simulink model "SimulinkOnramp"  (R2021a)
settings: Solver=VariableStepAuto  StartTime=0.0  StopTime=10.0  RelTol=1e-3
StartFcn:
  | learning.simulink.modelCallbacks.startFunction(gcs)
StopFcn:
  | learning.simulink.modelCallbacks.stopFunction(gcs)
model workspace (MAT data in the model file):
  courseObject.course = 'simulink'
  courseObject.chapter = 9
  courseObject.lesson = 1
  courseObject.section = 2
  courseObject.task = 1
  t_ans = [0; 0.25; 0.5; 0.75; 1; 1.25; 1.5; 1.75; 2; 2.25; 2.5; 2.75; 3; 3.25; 3.5; 3.75; 4; 4.25; 4.5; 4.75; 5; 5.25; 5.5; 5.75; 6; 6.25; 6.5; 6.75; 7; 7.25; 7.5; 7.75; 8; 8.25; 8.5; 8.75; 9; 9.25; 9.5; 9.75; 10]
  y_ans4 = [2.5; 5; 7.5; 10; 12.5; 15; 17.5; 20; 22.5; 25; 27.5; 30; 32.5; 35; 37.5; 40; 42.5; 45; 47.5; 50; 52.5; 55; 57.5; 60; 62.5; 65; 67.5; 70; 72.5; 75; 77.5; 80; 82.5; 85; 87.5; 90; 92.5; 95; 97.5; 100; 102.5]
  y_ans5 = [7.5; 10; 12.5; 15; 17.5; 20; 22.5; 25; 27.5; 30; 32.5; 35; 37.5; 40; 42.5; 45; 47.5; 50; 52.5; 55; 57.5; 60; 62.5; 65; 67.5; 70; 72.5; 75; 77.5; 80; 82.5; 85; 87.5; 90; 92.5; 95; 97.5; 100; 102.5; 105; 107.5]
libraries: signalChecks x1
CloseFcn:
  | learning.simulink.cleanupOnlineTraining
settings Model: Creator=HP  LastModifiedBy=HP
settings DataIOCC: SaveTime=off

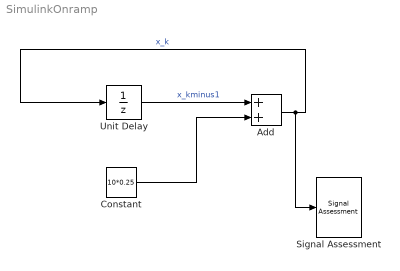
== system SimulinkOnramp ==
  Add : Sum
  Constant : Constant  Value=10*0.25
  Signal Assessment : signalChecks/Signal Assessment  signal_type='signal'  t_ans=t_ans  y_ans_upper=y_ans5  y_ans_lower=0  range=.005  rate_type=1  lesson=0  task=5  pass=1
  Unit Delay : UnitDelay  InitialCondition=5  SampleTime=0.25  HasFrameUpgradeWarning=on
  wires:
  Unit Delay/1 -> Add/1  "x_kminus1"
  Add/1 -> Signal Assessment/1, Unit Delay/1  "x_k"
  Constant/1 -> Add/2
